simulink model "costas_2"  (Simulink 3.00)
settings: Solver=ode5  SolverMode=SingleTasking  StartTime=0.0  StopTime=10.0  FixedStep=1/(5*1000)  RelTol=1e-3  AbsTol=1e-6
values from neighbouring files (symbols this model uses):
  f0 = 500    [chirp_1.m]    (also in costas1f.m = pf0; op_freq.m = 15; pll_5f.m = f01)
  kvco = pkvco    [costas1f.m]    (also in pll_5f.m = kvco1)
  tau = ptau    [costas1f.m]    (also in op_freq.m = 0.0106103295395; pll_5f.m = tau1)
  tau1 = ptau1    [costas1f.m]
  tau2 = ptau2    [costas1f.m]
settings Model: LimitMaxRows=on  MaxRows=5000

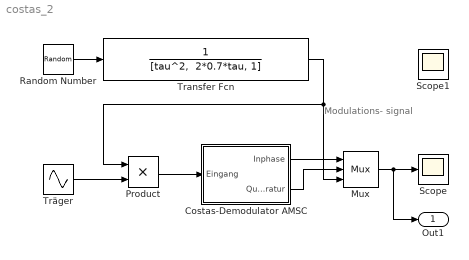
== system costas_2 ==
  note: Modulations-
      | signal
  Costas-Demodulator AMSC : Subsystem
  Mux : Mux  Inputs=3
      settings: DisplayOption=none
  Product : Product  Inputs=2  SaturateOnIntegerOverflow=on
  Random Number : RandomNumber  Mean=0  Variance=1  Seed=0  SampleTime=0
  Scope : Scope
      settings: TickLabels=on  TimeRange=0.1  YMin=-0.4  YMax=0.5  SaveToWorkspace=off  SaveName=ScopeData  DataFormat=Matrix
  Scope1 : Scope
      settings: Floating=on  TickLabels=on  TimeRange=0.1  YMin=-0.3  YMax=0.3  SaveToWorkspace=off  SaveName=ScopeData  DataFormat=Matrix
  Transfer Fcn : TransferFcn  Numerator=[1]  Denominator="[tau^2,  2*0.7*tau, 1]"
  Träger : Sin  Amplitude=1  Frequency=2*pi*f0  Phase=0  SampleTime=0
  Out1 : Outport  Port=1
  wires:
  Random Number/1 -> Transfer Fcn/1
  Transfer Fcn/1 -> Mux/3, Product/1
  Träger/1 -> Product/2
  Costas-Demodulator AMSC/1(Inphase) -> Mux/1
  Costas-Demodulator AMSC/2(Quadratur) -> Mux/2
  Mux/1 -> Scope/1, Out1/1
  Product/1 -> Costas-Demodulator AMSC/1(Eingang)

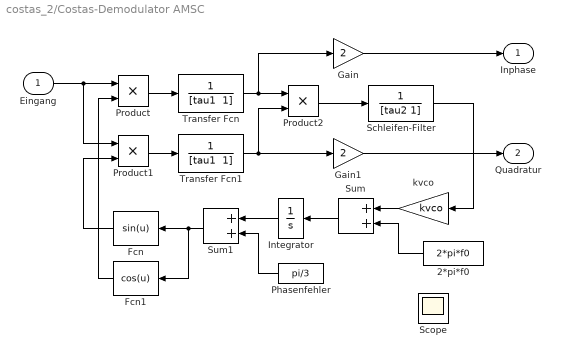
== system costas_2/Costas-Demodulator AMSC ==
  Eingang : Inport  Port=1  PortWidth=-1  SampleTime=-1  DataType=auto
      settings: SignalType=auto
  2*pi*f0 : Constant  Orientation=left  Value=2*pi*f0
  Fcn : Fcn  Orientation=left  Expr=sin(u)
  Fcn1 : Fcn  Orientation=left  Expr=cos(u)
  Gain : Gain  Gain=2  SaturateOnIntegerOverflow=on
  Gain1 : Gain  Gain=2  SaturateOnIntegerOverflow=on
  Integrator : Integrator  Orientation=left  ExternalReset=none  InitialConditionSource=internal  InitialCondition=0  LimitOutput=off  UpperSaturationLimit=inf  LowerSaturationLimit=-inf  ShowSaturationPort=off  ShowStatePort=off  AbsoluteTolerance=auto
  Phasenfehler : Constant  Orientation=left  Value=pi/3
  Product : Product  Inputs=2  SaturateOnIntegerOverflow=on
  Product1 : Product  Inputs=2  SaturateOnIntegerOverflow=on
  Product2 : Product  Inputs=2  SaturateOnIntegerOverflow=on
  Schleifen-Filter : TransferFcn  Numerator=[1]  Denominator=[tau2 1]
  Scope : Scope
      settings: Floating=on  TickLabels=on  TimeRange=0.1  YMin=-0.125  YMax=0.2  SaveToWorkspace=off  SaveName=ScopeData  DataFormat=Matrix
  Sum : Sum  Orientation=left  Inputs=++  SaturateOnIntegerOverflow=on
  Sum1 : Sum  Orientation=left  Inputs=++  SaturateOnIntegerOverflow=on
  Transfer Fcn : TransferFcn  Numerator=[1]  Denominator="[tau1  1]"
  Transfer Fcn1 : TransferFcn  Numerator=[1]  Denominator="[tau1  1]"
  kvco : Gain  Orientation=left  Gain=kvco  SaturateOnIntegerOverflow=on
  Inphase : Outport  Port=1
  Quadratur : Outport  Port=2
  wires:
  Eingang/1 -> Product/1, Product1/1
  Sum/1 -> Integrator/1
  2*pi*f0/1 -> Sum/2
  kvco/1 -> Sum/1
  Integrator/1 -> Sum1/1
  Phasenfehler/1 -> Sum1/2
  Product/1 -> Transfer Fcn/1
  Product1/1 -> Transfer Fcn1/1
  Product2/1 -> Schleifen-Filter/1
  Schleifen-Filter/1 -> kvco/1
  Fcn/1 -> Product1/2
  Sum1/1 -> Fcn/1, Fcn1/1
  Fcn1/1 -> Product/2
  Transfer Fcn/1 -> Product2/1, Gain/1
  Gain/1 -> Inphase/1
  Transfer Fcn1/1 -> Product2/2, Gain1/1
  Gain1/1 -> Quadratur/1
